simulink model "AddN4a_Model"  (R2024b)
settings: Solver=VariableStepAuto  StartTime=0.0  StopTime=10.0  RelTol=1e-3
libraries: NSA_DEVS_SOURCES x4, NSA_DEVS_MATH_OPERATIONS x1, NSA_DEVS_SINKS x1
settings Model: Creator=peter  LastModifiedBy=peter

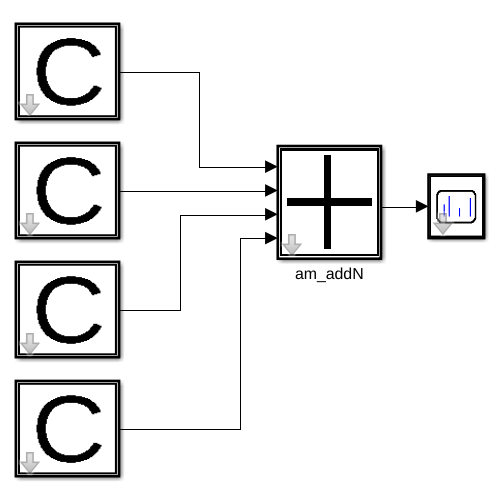
[thumbnail: Simulink's stored preview of the top-level diagram]
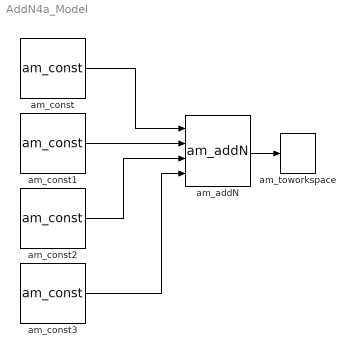
== system AddN4a_Model ==
  am_addN : NSA_DEVS_MATH_OPERATIONS/am_addN  N=4  tau=[0,1]  debug=0
      settings: SourceProductName=Math Operations
  am_const : NSA_DEVS_SOURCES/am_const  value=1  sendTime=[1,0]  debug=0
      settings: SourceProductName=Sources
  am_const1 : NSA_DEVS_SOURCES/am_const  value=2  sendTime=[2,0]  debug=0
      settings: SourceProductName=Sources
  am_const2 : NSA_DEVS_SOURCES/am_const  value=3  sendTime=[2,0]  debug=0
      settings: SourceProductName=Sources
  am_const3 : NSA_DEVS_SOURCES/am_const  value=4  sendTime=[2,0]  debug=0
      settings: SourceProductName=Sources
  am_toworkspace : NSA_DEVS_SINKS/am_toworkspace  varname="\"sum\""  t0=0  format="\"vector\""  tau=[0,5]  debug=0
      settings: SourceProductName=Sinks
  wires:
  am_addN/1 -> am_toworkspace/1
  am_const/1 -> am_addN/1
  am_const3/1 -> am_addN/4
  am_const2/1 -> am_addN/3
  am_const1/1 -> am_addN/2
